simulink model "IdqMap"  (R2022b)
settings: Solver=FixedStepDiscrete  StartTime=0.0  StopTime=10.0  FixedStep=0.0001  RelTol=1e-3
values from neighbouring files (symbols this model uses):
  RPM_CELL = 0.0    [MCU_IdqMap.sldd]
  TOR_CELL = 0.0    [MCU_IdqMap.sldd]
undefined symbols (not defined in the file or in its folder): ParamCfg_BaseUdc_u16, ParamCfg_IqMax_u16, ParamCfg_IqMin_u16, ParamCfg_MaxTorque_u16, ParamCfg_SpeedMax_u16, ParamCfg_TorqlookupRpmStep_u16, ParamCfg_TorqlookupTorqStep_u16, ParamCfg_WeakCalcEnable_u16, ParamCfg_WeakIdMax_u16, ParamCfg_WeakIdMin_u16
libraries: simulink x7, YS_UserDefined_Library x4
settings Model: DataDictionary=MCU_IdqMap.sldd  Creator=ZYH  LastModifiedBy=ZYH
settings OptimizationCC: DefaultParameterBehavior=Inlined  EnhancedBackFolding=on  PassReuseOutputArgsAs=Individual arguments  ZeroExternalMemoryAtStartup=off  ZeroInternalMemoryAtStartup=off  OptimizeBlockOrder=speed  DifferentSizesBufferReuse=on  OptimizationCustomize=off  EfficientTunableParamExpr=on
settings DebuggingCC: ParameterTunabilityLossMsg=error
settings SFSimCC: MATLABDynamicMemAlloc=off
settings RTWCC: Description=Embedded Coder  SystemTargetFile=ert.tlc  GenCodeOnly=on  TemplateMakefile=ert_default_tmf
settings CodeAppCC: ForceParamTrailComments=on  IgnoreCustomStorageClasses=off  OperatorAnnotations=on  SimulinkDataObjDesc=on  SFDataObjDesc=on  InsertBlockDesc=on
settings ERTTargetCC: TargetLangStandard=C99 (ISO)  GenerateSampleERTMain=on  InlinedParameterPlacement=NonHierarchical  ERTCustomFileTemplate=example_file_process.tlc

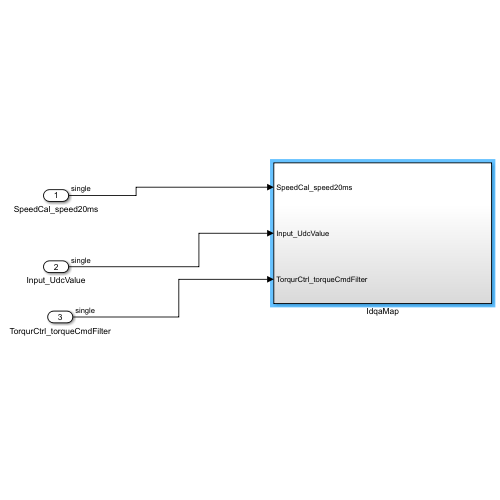
[thumbnail: Simulink's stored preview of the top-level diagram]
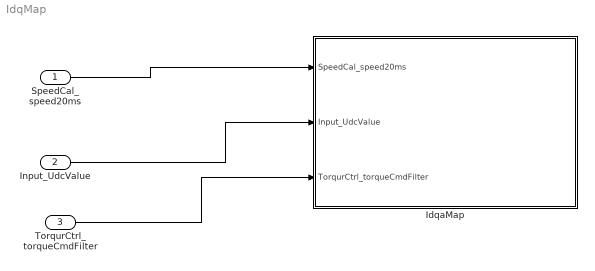
== system IdqMap ==
  SpeedCal_speed20ms : Inport
  Input_UdcValue : Inport  Port=2
  TorqurCtrl_torqueCmdFilter : Inport  Port=3
  IdqaMap : Subsystem
  wires:
  SpeedCal_speed20ms/1 -> IdqaMap/1(SpeedCal_speed20ms)
  Input_UdcValue/1 -> IdqaMap/2(Input_UdcValue)
  TorqurCtrl_torqueCmdFilter/1 -> IdqaMap/3(TorqurCtrl_torqueCmdFilter)

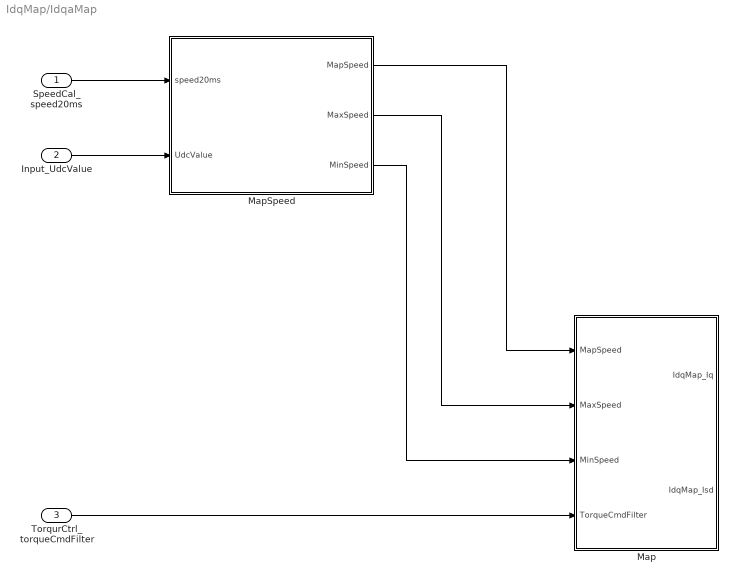
== system IdqMap/IdqaMap ==
  SpeedCal_speed20ms : Inport
  Input_UdcValue : Inport  Port=2
  TorqurCtrl_torqueCmdFilter : Inport  Port=3
  Map : Subsystem
  MapSpeed : Subsystem
  wires:
  SpeedCal_speed20ms/1 -> MapSpeed/1(speed20ms)
  Input_UdcValue/1 -> MapSpeed/2(UdcValue)
  MapSpeed/1(MapSpeed) -> Map/1(MapSpeed)
  TorqurCtrl_torqueCmdFilter/1 -> Map/4(TorqueCmdFilter)
  MapSpeed/2(MaxSpeed) -> Map/2(MaxSpeed)
  MapSpeed/3(MinSpeed) -> Map/3(MinSpeed)

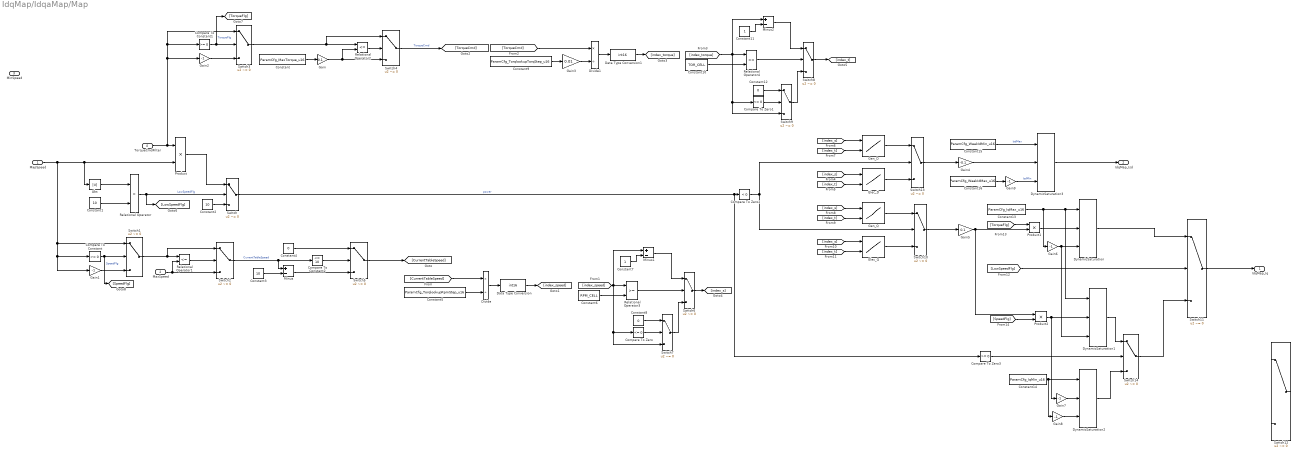
== system IdqMap/IdqaMap/Map ==
  MapSpeed : Inport
  MaxSpeed : Inport  Port=2
  MinSpeed : Inport  Port=3
  TorqueCmdFilter : Inport  Port=4
  Abs : Abs  SaturateOnIntegerOverflow=off
  Compare To Constant : simulink/Logic and Bit Operations/Compare To Constant  relop=>=  const=0  OutDataTypeStr=boolean
  Compare To Constant1 : simulink/Logic and Bit Operations/Compare To Constant  relop=>=  const=0  OutDataTypeStr=boolean
  Compare To Constant2 : simulink/Logic and Bit Operations/Compare To Constant  relop=<=  const=10  OutDataTypeStr=boolean
  Compare To Zero : simulink/Logic and Bit Operations/Compare To Zero  relop=<=  OutDataTypeStr=boolean
  Compare To Zero1 : simulink/Logic and Bit Operations/Compare To Zero  relop=<=  OutDataTypeStr=boolean
  Compare To Zero2 : simulink/Logic and Bit Operations/Compare To Zero  relop=<  OutDataTypeStr=boolean
  Compare To Zero3 : simulink/Logic and Bit Operations/Compare To Zero  relop=>=  OutDataTypeStr=boolean
  Constant : Constant  Value=ParamCfg_MaxTorque_u16
  Constant1 : Constant  Value=10  OutDataTypeStr=single
  Constant10 : Constant  Value=TOR_CELL
  Constant11 : Constant  OutDataTypeStr=int16
  Constant12 : Constant  Value=0  OutDataTypeStr=int16
  Constant13 : Constant  Value=ParamCfg_IqMax_u16  OutDataTypeStr=single
  Constant14 : Constant  Value=ParamCfg_IqMin_u16  OutDataTypeStr=single
  Constant15 : Constant  Value=ParamCfg_WeakIdMin_u16  OutDataTypeStr=single
  Constant16 : Constant  Value=ParamCfg_WeakIdMax_u16  OutDataTypeStr=single
  Constant2 : Constant  Value=10  OutDataTypeStr=single
  Constant3 : Constant  Value=10  OutDataTypeStr=single
  Constant4 : Constant  Value=0  OutDataTypeStr=single
  Constant5 : Constant  Value=ParamCfg_TorqlookupRpmStep_u16
  Constant6 : Constant  Value=RPM_CELL
  Constant7 : Constant  OutDataTypeStr=int16
  Constant8 : Constant  Value=0  OutDataTypeStr=int16
  Constant9 : Constant  Value=ParamCfg_TorqlookupTorqStep_u16
  Data Type Conversion : DataTypeConversion  OutDataTypeStr=int16  SaturateOnIntegerOverflow=off  RndMeth=Floor
  Data Type Conversion1 : DataTypeConversion  OutDataTypeStr=int16  SaturateOnIntegerOverflow=off  RndMeth=Floor
  Divide : Product  Inputs=*/
  Divide1 : Product  Inputs=*/
  DynamicSaturation{,1..3} (4 alike) : YS_UserDefined_Library/Saturation/DynamicSaturation
      settings: SourceProductName=YS
  Elec_D : Lookup_n-D  BreakpointsForDimension1=[1:3]  BreakpointsForDimension2=[1:3]  IndexSearchMethod=Linear search  ExtrapMethod=Clip  UseLastTableValue=on  InternalRulePriority=Speed  OutDataTypeStr=single  RndMeth=Simplest
      settings: InputPortMap=u0,u1
  Elec_Q : Lookup_n-D  BreakpointsForDimension1=[1:3]  BreakpointsForDimension2=[1:3]  IndexSearchMethod=Linear search  ExtrapMethod=Clip  UseLastTableValue=on  InternalRulePriority=Speed  RndMeth=Simplest
      settings: InputPortMap=u0,u1
  Gain : Gain  Gain=0.1  ParamDataTypeStr=single  OutDataTypeStr=single
  Gain{1..2,6..9} (6 alike) : Gain  Gain=-1  ParamDataTypeStr=single  OutDataTypeStr=single
  Gain3 : Gain  Gain=0.01  OutDataTypeStr=single
  Gain4 : Gain  Gain=-0.1  OutDataTypeStr=single
  Gain5 : Gain  Gain=0.1  OutDataTypeStr=single
  Gen_D : Lookup_n-D  BreakpointsForDimension1=[1:3]  BreakpointsForDimension2=[1:3]  IndexSearchMethod=Linear search  ExtrapMethod=Clip  InternalRulePriority=Speed  RndMeth=Simplest
      settings: InputPortMap=u0,u1
  Gen_Q : Lookup_n-D  BreakpointsForDimension1=[1:3]  BreakpointsForDimension2=[1:3]  IndexSearchMethod=Linear search  ExtrapMethod=Clip  UseLastTableValue=on  InternalRulePriority=Speed  RndMeth=Simplest
      settings: InputPortMap=u0,u1
  Minus : Sum  Inputs=+-
  Minus1 : Sum  Inputs=+-
  Minus2 : Sum  Inputs=+-
  Product : Product
  Product1 : Product
  Product2 : Product
  Relational Operator : RelationalOperator  Operator=>  OutDataTypeStr=boolean  RndMeth=Simplest  InputSameDT=off
  Relational Operator1 : RelationalOperator  Operator=<=  OutDataTypeStr=boolean  RndMeth=Simplest  InputSameDT=off
  Relational Operator2 : RelationalOperator  Operator=<=  OutDataTypeStr=boolean  RndMeth=Simplest  InputSameDT=off
  Relational Operator3 : RelationalOperator  OutDataTypeStr=boolean  RndMeth=Simplest  InputSameDT=off
  Relational Operator4 : RelationalOperator  OutDataTypeStr=boolean  RndMeth=Simplest  InputSameDT=off
  Switch{,1..14} (15 alike) : Switch  Criteria=u2 ~= 0  SaturateOnIntegerOverflow=off  InputSameDT=off
  IdqMap_Iq : Outport
  IdqMap_Isd : Outport  Port=2
  wires:
  MapSpeed/1 -> Switch1/1, Gain1/1, Compare To Constant/1, Abs/1, Product/2
  Constant/1 -> Gain/1
  Constant1/1 -> Relational Operator/2
  Abs/1 -> Relational Operator/1
  Relational Operator/1 -> [LowSpeedFlg], Switch/2  "LowSpeedFlg"
  Constant2/1 -> Switch/3
  Product/1 -> Switch/1
  Compare To Constant/1 -> [SpeedFlg], Switch1/2  "SpeedFlg"
  Gain1/1 -> Switch1/3
  Switch1/1 -> Switch2/1, Relational Operator1/1
  MaxSpeed/1 -> Switch2/3, Relational Operator1/2
  Relational Operator1/1 -> Switch2/2
  TorqueCmdFilter/1 -> Switch3/1, Compare To Constant1/1, Gain2/1, Product/1
  Compare To Constant1/1 -> [TorqueFlg], Switch3/2  "TorqueFlg"
  Gain2/1 -> Switch3/3
  Switch3/1 -> Switch4/1, Relational Operator2/1
  Gain/1 -> Switch4/3, Relational Operator2/2
  Relational Operator2/1 -> Switch4/2
  Switch2/1 -> Minus/1, Compare To Constant2/1  "CurrentTableSpeed"
  Switch4/1 -> [TorqueCmd]  "TorqueCmd"
  Compare To Constant2/1 -> Switch5/2
  Constant3/1 -> Minus/2
  Minus/1 -> Switch5/3
  Constant4/1 -> Switch5/1
  Switch5/1 -> [CurrentTableSpeed]
  [CurrentTableSpeed] -> Divide/1
  Constant5/1 -> Divide/2
  Divide/1 -> Data Type Conversion/1
  Data Type Conversion/1 -> [index_speed]
  [index_speed] -> Switch7/3, Compare To Zero/1, Relational Operator3/1, Minus1/1
  Constant6/1 -> Relational Operator3/2
  Relational Operator3/1 -> Switch6/2
  Minus1/1 -> Switch6/1
  Constant7/1 -> Minus1/2
  Compare To Zero/1 -> Switch7/2
  Constant8/1 -> Switch7/1
  Switch7/1 -> Switch6/3
  Constant9/1 -> Gain3/1
  [TorqueCmd] -> Divide1/1
  Gain3/1 -> Divide1/2
  Divide1/1 -> Data Type Conversion1/1
  Minus2/1 -> Switch8/1
  Constant10/1 -> Relational Operator4/2
  Relational Operator4/1 -> Switch8/2
  [index_torque] -> Switch9/3, Compare To Zero1/1, Minus2/1, Relational Operator4/1
  Constant11/1 -> Minus2/2
  Constant12/1 -> Switch9/1
  Compare To Zero1/1 -> Switch9/2
  Switch9/1 -> Switch8/3
  Switch6/1 -> [index_s]
  Switch8/1 -> [index_t]
  Data Type Conversion1/1 -> [index_torque]
  [index_t] -> Elec_D/2
  [index_s] -> Elec_D/1
  Switch/1 -> Compare To Zero3/1, Compare To Zero2/1  "power"
  Compare To Zero2/1 -> Switch10/2, Switch13/2
  Elec_D/1 -> Switch13/3
  Elec_Q/1 -> Switch10/3
  Gen_D/1 -> Switch13/1
  Gen_Q/1 -> Switch10/1
  Switch13/1 -> Gain4/1
  Switch10/1 -> Gain5/1
  [index_s] -> Gen_D/1
  [index_t] -> Gen_D/2
  [index_s] -> Elec_Q/1
  [index_t] -> Elec_Q/2
  [index_s] -> Gen_Q/1
  [index_t] -> Gen_Q/2
  [LowSpeedFlg] -> Switch11/2
  [TorqueFlg] -> Product1/1
  Gain5/1 -> Product2/1, Product1/2
  Product1/1 -> DynamicSaturation/2
  Constant13/1 -> Gain6/1, DynamicSaturation1/1, DynamicSaturation/1
  Gain6/1 -> DynamicSaturation1/3, DynamicSaturation/3
  DynamicSaturation/1 -> Switch11/1
  [SpeedFlg] -> Product2/2
  Compare To Zero3/1 -> Switch14/2
  DynamicSaturation1/1 -> Switch14/1
  Product2/1 -> Gain7/1, DynamicSaturation1/2
  DynamicSaturation2/1 -> Switch14/3
  Gain7/1 -> DynamicSaturation2/2
  Switch14/1 -> Switch11/3
  Constant14/1 -> Gain8/1, DynamicSaturation2/1
  Gain8/1 -> DynamicSaturation2/3
  Switch11/1 -> IdqMap_Iq/1
  Gain4/1 -> DynamicSaturation3/2
  Constant15/1 -> DynamicSaturation3/1  "IsdMax"
  Gain9/1 -> DynamicSaturation3/3  "IsdMin"
  Constant16/1 -> Gain9/1
  DynamicSaturation3/1 -> IdqMap_Isd/1

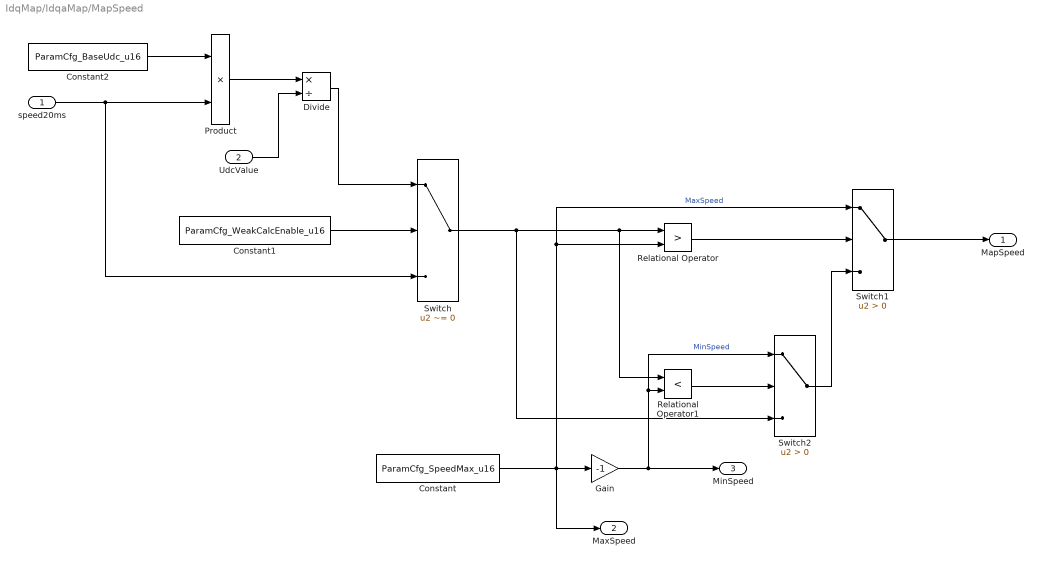
== system IdqMap/IdqaMap/MapSpeed ==
  speed20ms : Inport
  UdcValue : Inport  Port=2
  Constant : Constant  Value=ParamCfg_SpeedMax_u16
  Constant1 : Constant  Value=ParamCfg_WeakCalcEnable_u16
  Constant2 : Constant  Value=ParamCfg_BaseUdc_u16
  Divide : Product  Inputs=*/  OutDataTypeStr=single
  Gain : Gain  Gain=-1  ParamDataTypeStr=single  OutDataTypeStr=single
  Product : Product
  Relational Operator : RelationalOperator  Operator=>  OutDataTypeStr=boolean  RndMeth=Simplest  InputSameDT=off
  Relational Operator1 : RelationalOperator  Operator=<  OutDataTypeStr=boolean  RndMeth=Simplest  InputSameDT=off
  Switch : Switch  Criteria=u2 ~= 0  SaturateOnIntegerOverflow=off  InputSameDT=off
  Switch1 : Switch  Criteria=u2 > Threshold  SaturateOnIntegerOverflow=off  InputSameDT=off
  Switch2 : Switch  Criteria=u2 > Threshold  SaturateOnIntegerOverflow=off  InputSameDT=off
  MapSpeed : Outport
  MaxSpeed : Outport  Port=2
  MinSpeed : Outport  Port=3
  wires:
  Constant/1 -> MaxSpeed/1, Gain/1, Relational Operator/2, Switch1/1  "MaxSpeed"
  Divide/1 -> Switch/1
  Constant1/1 -> Switch/2
  Product/1 -> Divide/1
  UdcValue/1 -> Divide/2
  Constant2/1 -> Product/1
  speed20ms/1 -> Switch/3, Product/2
  Switch/1 -> Switch2/3, Relational Operator1/1, Relational Operator/1
  Relational Operator/1 -> Switch1/2
  Gain/1 -> MinSpeed/1, Switch2/1, Relational Operator1/2  "MinSpeed"
  Relational Operator1/1 -> Switch2/2
  Switch2/1 -> Switch1/3
  Switch1/1 -> MapSpeed/1
